simulink library "libH7_3DOF"  (R2021b)
settings: Solver=VariableStepAuto  StartTime=0.0  StopTime=10.0  RelTol=1e-3
undefined symbols (not defined in the file or in its folder): initial_conds, pod
libraries: $bdroot x1
settings Model: Creator=Ferran  LastModifiedBy=Ferran

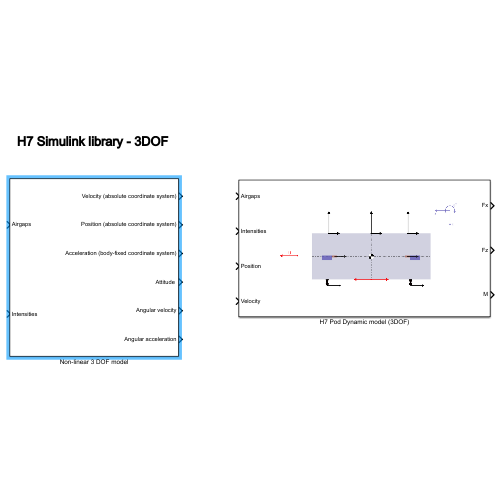
[thumbnail: Simulink's stored preview of the top-level diagram]
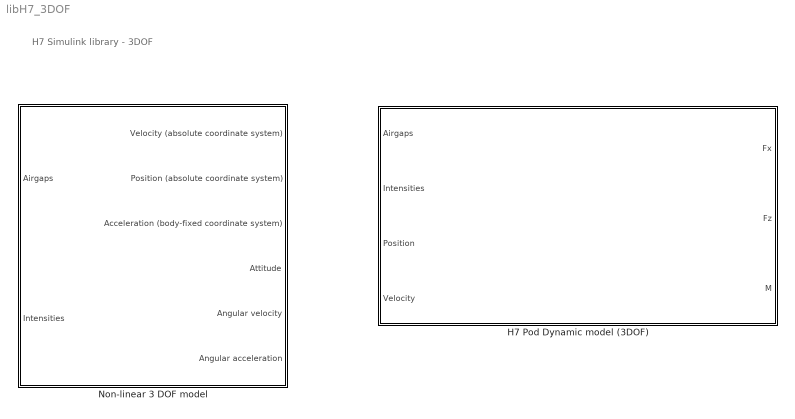
== system libH7_3DOF ==
  note: H7 Simulink library - 3DOF
  H7 Pod Dynamic model (3DOF) : Subsystem
      mask Display: image('FBD_2D.png', [0.12 0.12 0.78 0.78]); % Use "Edit Image" on toolstrip to change.
  Non-linear 3 DOF model : Subsystem

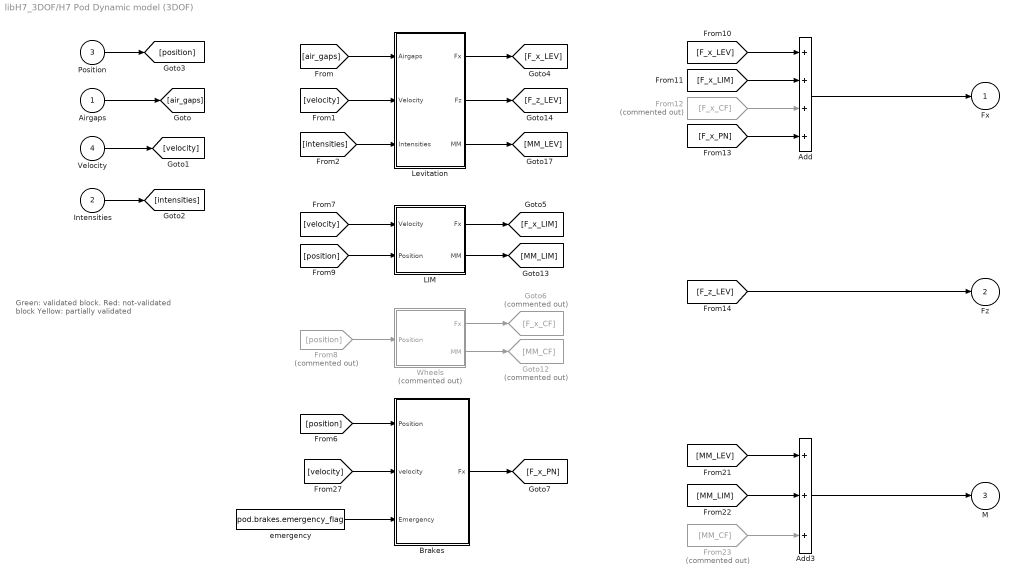
== system libH7_3DOF/H7 Pod Dynamic model (3DOF) ==
  note: Green: validated block.
      | Red: not-validated block
      | Yellow: partially validated
  Airgaps : Inport
  Intensities : Inport  Port=2
  Position : Inport  Port=3
  Velocity : Inport  Port=4
  Add : Sum  Inputs=++++
  Add3 : Sum  Inputs=+++
  "Brakes " : Subsystem  AncestorBlock=libH7/H7 Pod Dynamic model/Brakes
  From12 : From  Commented=on  GotoTag=F_x_CF
  From23 : From  Commented=on  GotoTag=MM_CF
  From8 : From  Commented=on  GotoTag=position
  Goto12 : Goto  Commented=on  GotoTag=MM_CF
  Goto6 : Goto  Commented=on  GotoTag=F_x_CF
  "LIM " : Subsystem  AncestorBlock=libH7/H7 Pod Dynamic model/LIM
  "Levitation " : Subsystem  AncestorBlock=libH7/H7 Pod Dynamic model/Levitation
  "Wheels " : Subsystem  Commented=on  AncestorBlock=libH7/H7 Pod Dynamic model/Wheels
  emergency : Constant  Value=pod.brakes.emergency_flag
  Fx : Outport
  Fz : Outport  Port=2
  M : Outport  Port=3
  wires:
  "Wheels "/2(MM) -> Goto12/1
  "Wheels "/1(Fx) -> Goto6/1
  [velocity] -> "LIM "/1(Velocity)
  [position] -> "Brakes "/1(Position)
  [intensities] -> "Levitation "/3(Intensities)
  [MM_LIM] -> Add3/2
  [velocity] -> "Brakes "/2(velocity)
  Velocity/1 -> [velocity]
  Add3/1 -> M/1
  [velocity] -> "Levitation "/2(Velocity)
  Position/1 -> [position]
  Airgaps/1 -> [air_gaps]
  From8/1 -> "Wheels "/1(Position)
  From23/1 -> Add3/3
  Add/1 -> Fx/1
  [F_x_LIM] -> Add/2
  "Brakes "/1(Fx) -> [F_x_PN]
  [F_x_PN] -> Add/4
  Intensities/1 -> [intensities]
  [F_x_LEV] -> Add/1
  [F_z_LEV] -> Fz/1
  [MM_LEV] -> Add3/1
  "Levitation "/3(MM) -> [MM_LEV]
  [position] -> "LIM "/2(Position)
  "LIM "/2(MM) -> [MM_LIM]
  From12/1 -> Add/3
  "Levitation "/1(Fx) -> [F_x_LEV]
  [air_gaps] -> "Levitation "/1(Airgaps)
  "LIM "/1(Fx) -> [F_x_LIM]
  emergency/1 -> "Brakes "/3(Emergency)
  "Levitation "/2(Fz) -> [F_z_LEV]

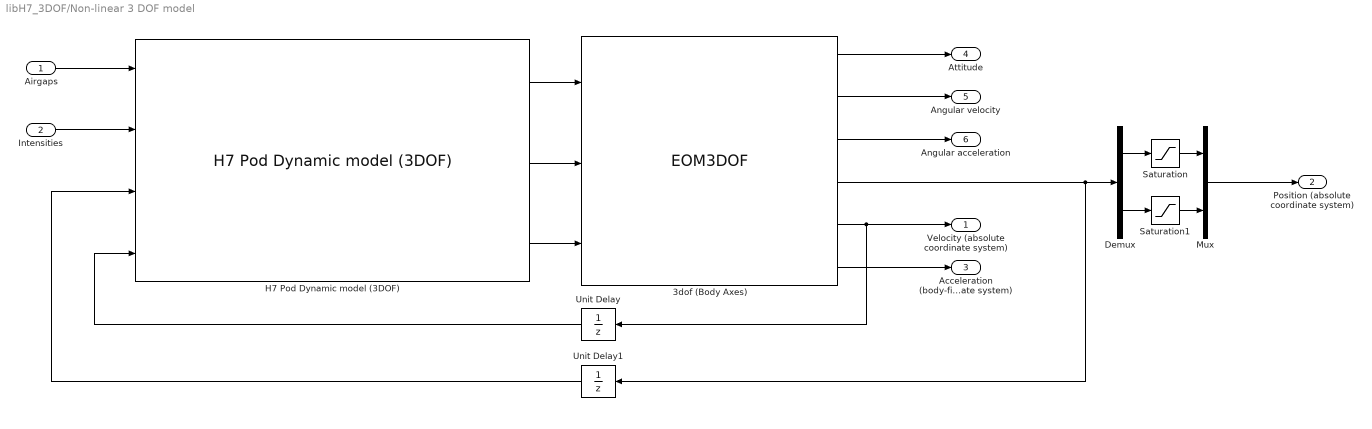
== system libH7_3DOF/Non-linear 3 DOF model ==
  Airgaps : Inport
  Intensities : Inport  Port=2
  3dof (Body Axes) : EOM3DOF  v_ini=1e-10  theta_ini=initial_conds.ang_0(2)  q_ini=initial_conds.w_0(2)  pos_ini=initial_conds.x_0(1:2:3)  mass=pod.mass.mass  Iyy=pod.mass.inertia(2,2)
  Demux : Demux  Outputs=2
  H7 Pod Dynamic model (3DOF) : $bdroot/H7 Pod Dynamic model (3DOF)  SystemSampleTime=-1  VariantActivationTime=update diagram  Latency=0  AutoFrameSizeCalculation=off
  Mux : Mux  Inputs=2
  Saturation : Saturate  UpperLimit=20  LowerLimit=0
  Saturation1 : Saturate  UpperLimit=pod.geometry.z_LEV + 0.023  LowerLimit=pod.geometry.z_LEV + 0.012
  Unit Delay : UnitDelay  InitialCondition=[0,0]  SampleTime=-1  HasFrameUpgradeWarning=on
  Unit Delay1 : UnitDelay  InitialCondition=initial_conds.x_0(1:2:3)  SampleTime=-1  HasFrameUpgradeWarning=on
  Velocity (absolute coordinate system) : Outport
  Position (absolute coordinate system) : Outport  Port=2
  Acceleration (body-fixed coordinate system) : Outport  Port=3
  "Attitude " : Outport  Port=4
  Angular velocity : Outport  Port=5
  Angular acceleration : Outport  Port=6
  wires:
  H7 Pod Dynamic model (3DOF)/1 -> 3dof (Body Axes)/1
  3dof (Body Axes)/2 -> Angular velocity/1
  H7 Pod Dynamic model (3DOF)/3 -> 3dof (Body Axes)/3
  H7 Pod Dynamic model (3DOF)/2 -> 3dof (Body Axes)/2
  Intensities/1 -> H7 Pod Dynamic model (3DOF)/2
  Airgaps/1 -> H7 Pod Dynamic model (3DOF)/1
  3dof (Body Axes)/6 -> Acceleration (body-fixed coordinate system)/1
  3dof (Body Axes)/3 -> Angular acceleration/1
  3dof (Body Axes)/5 -> Velocity (absolute coordinate system)/1, Unit Delay/1
  3dof (Body Axes)/4 -> Demux/1, Unit Delay1/1
  3dof (Body Axes)/1 -> "Attitude "/1
  Demux/1 -> Saturation/1
  Demux/2 -> Saturation1/1
  Mux/1 -> Position (absolute coordinate system)/1
  Unit Delay/1 -> H7 Pod Dynamic model (3DOF)/4
  Unit Delay1/1 -> H7 Pod Dynamic model (3DOF)/3
  Saturation/1 -> Mux/1
  Saturation1/1 -> Mux/2

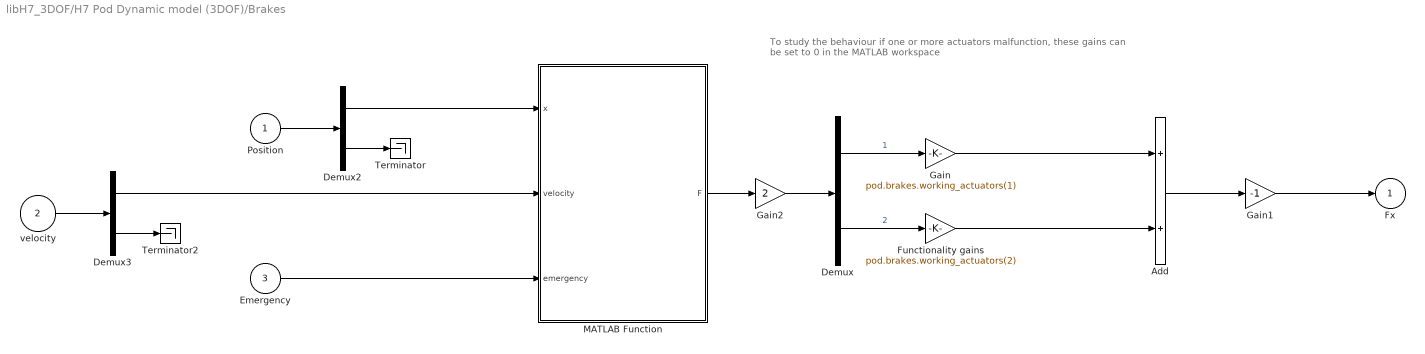
== system libH7_3DOF/H7 Pod Dynamic model (3DOF)/Brakes  ==
  note: To study the behaviour if one or more actuators malfunction,
      | these gains can be set to 0 in the MATLAB workspace
  Position : Inport
  velocity : Inport  Port=2
  Emergency : Inport  Port=3
  Add : Sum
  Demux : Demux  Outputs=2
  Demux2 : Demux  Outputs=2
  Demux3 : Demux  Outputs=2
  Functionality gains : Gain  Gain=pod.brakes.working_actuators(2)
  Gain : Gain  Gain=pod.brakes.working_actuators(1)
  Gain1 : Gain  Gain=-1
  Gain2 : Gain  Gain=2
  MATLAB Function : MATLAB Function  TreatAsAtomicUnit=on
  Terminator : Terminator
  Terminator2 : Terminator
  Fx : Outport
  wires:
  Demux3/1 -> MATLAB Function/2(velocity)
  Demux3/2 -> Terminator2/1
  velocity/1 -> Demux3/1
  Demux2/2 -> Terminator/1
  Demux2/1 -> MATLAB Function/1(x)
  Position/1 -> Demux2/1
  Gain/1 -> Add/1
  Functionality gains/1 -> Add/2
  Demux/2 -> Functionality gains/1  "2"
  Demux/1 -> Gain/1  "1"
  MATLAB Function/1(F) -> Gain2/1
  Emergency/1 -> MATLAB Function/3(emergency)
  Gain2/1 -> Demux/1
  Add/1 -> Gain1/1
  Gain1/1 -> Fx/1

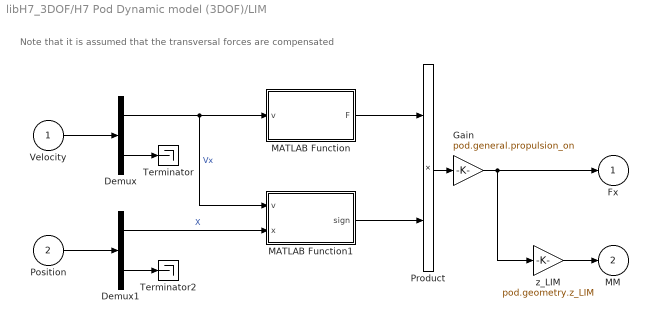
== system libH7_3DOF/H7 Pod Dynamic model (3DOF)/LIM  ==
  note: Note that it is assumed that the transversal forces are compensated
  Velocity : Inport
  Position : Inport  Port=2
  Demux : Demux  Outputs=2
  Demux1 : Demux  Outputs=2
  Gain : Gain  Gain=pod.general.propulsion_on
  MATLAB Function : MATLAB Function  TreatAsAtomicUnit=on
  MATLAB Function1 : MATLAB Function  TreatAsAtomicUnit=on
  Product : Product
  Terminator : Terminator
  Terminator2 : Terminator
  z_LIM : Gain  Gain=pod.geometry.z_LIM
  Fx : Outport
  MM : Outport  Port=2
  wires:
  z_LIM/1 -> MM/1
  Product/1 -> Gain/1
  MATLAB Function/1(F) -> Product/1
  MATLAB Function1/1(sign) -> Product/2
  Demux1/1 -> MATLAB Function1/2(x)  "X"
  Demux1/2 -> Terminator2/1
  Position/1 -> Demux1/1
  Demux/1 -> MATLAB Function1/1(v), MATLAB Function/1(v)  "Vx"
  Demux/2 -> Terminator/1
  Velocity/1 -> Demux/1
  Gain/1 -> Fx/1, z_LIM/1

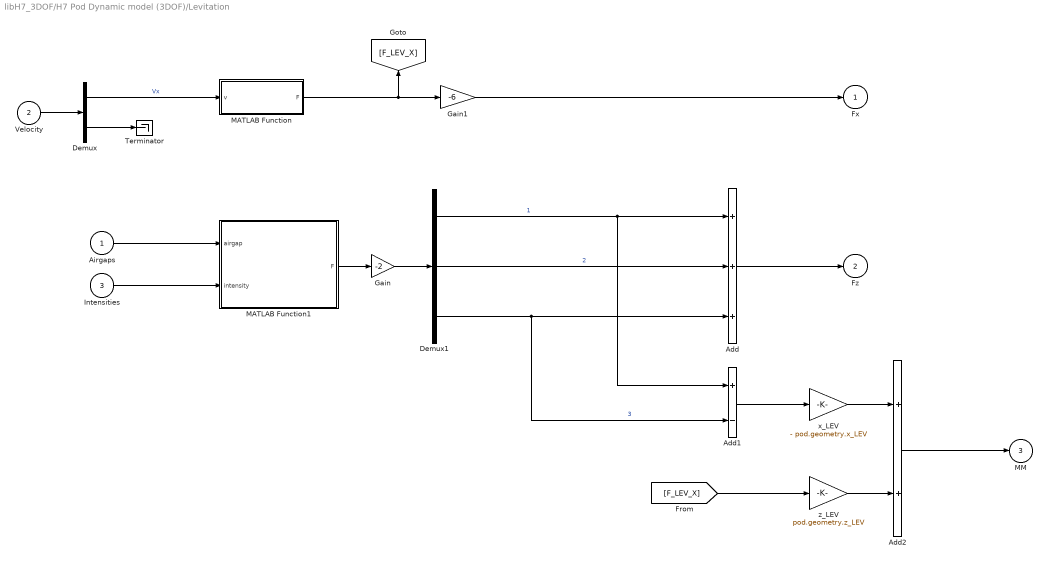
== system libH7_3DOF/H7 Pod Dynamic model (3DOF)/Levitation  ==
  Airgaps : Inport
  Velocity : Inport  Port=2
  Intensities : Inport  Port=3
  Add : Sum  Inputs=+++
  Add1 : Sum  Inputs=+-
  Add2 : Sum
  Demux : Demux  Outputs=2
  Demux1 : Demux  Outputs=3
  Gain : Gain  Gain=-2
  Gain1 : Gain  Gain=-6
  MATLAB Function : MATLAB Function  TreatAsAtomicUnit=on
  MATLAB Function1 : MATLAB Function  TreatAsAtomicUnit=on
  Terminator : Terminator
  x_LEV : Gain  Gain=- pod.geometry.x_LEV
  z_LEV : Gain  Gain=pod.geometry.z_LEV
  Fx : Outport
  Fz : Outport  Port=2
  MM : Outport  Port=3
  wires:
  MATLAB Function/1(F) -> Gain1/1, [F_LEV_X]
  Gain1/1 -> Fx/1
  MATLAB Function1/1(F) -> Gain/1
  Intensities/1 -> MATLAB Function1/2(intensity)
  Airgaps/1 -> MATLAB Function1/1(airgap)
  Demux/1 -> MATLAB Function/1(v)  "Vx"
  Velocity/1 -> Demux/1
  Demux/2 -> Terminator/1
  Gain/1 -> Demux1/1
  Demux1/2 -> Add/2  "2"
  Demux1/3 -> Add1/2, Add/3  "3"
  Demux1/1 -> Add1/1, Add/1  "1"
  Add/1 -> Fz/1
  Add1/1 -> x_LEV/1
  [F_LEV_X] -> z_LEV/1
  z_LEV/1 -> Add2/2
  x_LEV/1 -> Add2/1
  Add2/1 -> MM/1

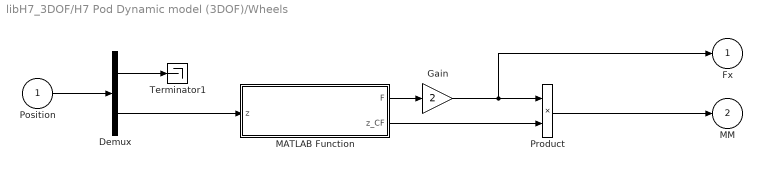
== system libH7_3DOF/H7 Pod Dynamic model (3DOF)/Wheels  ==
  Position : Inport
  Demux : Demux  Outputs=2
  Gain : Gain  Gain=2
  MATLAB Function : MATLAB Function  TreatAsAtomicUnit=on
  Product : Product
  Terminator1 : Terminator
  Fx : Outport
  MM : Outport  Port=2
  wires:
  Product/1 -> MM/1
  MATLAB Function/2(z_CF) -> Product/2
  Demux/1 -> Terminator1/1
  MATLAB Function/1(F) -> Gain/1
  Demux/2 -> MATLAB Function/1(z)
  Position/1 -> Demux/1
  Gain/1 -> Product/1, Fx/1

== matlab function libH7_3DOF/H7 Pod Dynamic model (3DOF)/Brakes /MATLAB Function ==
  data: x input; velocity input; F output; emergency input; pod parameter
function F  = brakes_activation(x, velocity, emergency, pod)
% Computes the braking force of the pneumatic actuators if and only if 
%     (1) The emergency flag has been raised
%     (2) The pod is above the acceleration phase distance
% ═════════════════════════════════════════════════════════════════════════
% Last updated: 20.12.2021
% ═════════════════════════════════════════════════════════════════════════

num_brakes = pod.brakes.n / 2;

if (emergency == 1 && x >= pod.brakes.d && velocity >= 0)
    F       = pod.brakes.force * ones(num_brakes,1);
else
    F       = zeros(num_brakes,1);
end

== matlab function libH7_3DOF/H7 Pod Dynamic model (3DOF)/LIM /MATLAB Function ==
  data: v input; F output; pod parameter
function F = LIMtraction(v, pod)
% Computes the traction force (N) of the LIM as a function of 
% the absolute velocity of the prototype (m/s)
% ═════════════════════════════════════════════════════════════════════════
% Last updated: 20.12.2021
% ═════════════════════════════════════════════════════════════════════════

F = pod.propulsion.poly.p3*v^3 + ...
    pod.propulsion.poly.p2*v^2 + ...
    pod.propulsion.poly.p1*v   + ...
    pod.propulsion.poly.p0;

== matlab function libH7_3DOF/H7 Pod Dynamic model (3DOF)/LIM /MATLAB Function1 ==
  data: v input; x input; sign output; pod parameter
function sign = LIMdirection(v, x, pod)
% Decides if the LIM force is being applied to accelerate or to brake 
% by comparing the position of the pod with a predefined treshold
% ═════════════════════════════════════════════════════════════════════════
% Last updated: 20.12.2021
% ═════════════════════════════════════════════════════════════════════════

if x >= pod.brakes.d && v > 0    
    sign = -1;
elseif x >= pod.brakes.d && v <= 0
    sign = 0;
else
    sign = 1;
end

== matlab function libH7_3DOF/H7 Pod Dynamic model (3DOF)/Levitation /MATLAB Function ==
  data: v input; F output; pod parameter
function F = HEMSdrag(v, pod)
% Computes the drag force (N) of one HEMS unit as a function of the 
% velocity (m/s)
% ═════════════════════════════════════════════════════════════════════════
% Last updated: 16.01.2022
% ═════════════════════════════════════════════════════════════════════════

if v < 1e-3
    v = 0;
end

F = pod.levitation.drag_1_unit.poly.p3*v^3 + ...
    pod.levitation.drag_1_unit.poly.p2*v^2 + ...
    pod.levitation.drag_1_unit.poly.p1*v   + ...
    pod.levitation.drag_1_unit.poly.p0;

== matlab function libH7_3DOF/H7 Pod Dynamic model (3DOF)/Levitation /MATLAB Function1 ==
  data: airgap input; F output; intensity input; pod parameter
function F = HEMSlev(airgap, intensity, pod)
% Computes the levitation force (N) of all the HEMS units as a function of 
% their air gaps (mm) and intensities (A)
% ═════════════════════════════════════════════════════════════════════════
% Last updated: 15.12.2021
% ════════════════════════════════════════════════════════════════════════

x   = airgap;
y   = intensity;

F = pod.levitation.poly_1_unit.p00 + ...
    pod.levitation.poly_1_unit.p10.*x + ...
    pod.levitation.poly_1_unit.p01.*y + ...
    pod.levitation.poly_1_unit.p20.*x.^2 + ...
    pod.levitation.poly_1_unit.p11.*x.*y + ...
    pod.levitation.poly_1_unit.p02.*y.^2 + ...
    pod.levitation.poly_1_unit.p21.*x.^2.*y + ...
    pod.levitation.poly_1_unit.p12.*x.*y.^2 + ...
    pod.levitation.poly_1_unit.p03.*y.^3;

== matlab function libH7_3DOF/H7 Pod Dynamic model (3DOF)/Wheels /MATLAB Function ==
  data: z input; F output; pod parameter; z_CF output
function [F, z_CF] = rollingFriction(z, pod)
% Computes the rolling resistance force (N) of the wheels. It distinguishes
% 3 cases: 
%   (1) z = 0. Pod touching the ground
%   (2) z = z_max. Pod touching the ceiling. It is assumed no current
%   applied to the HEMS. 
%   (3) Otherwise. Pod levitating. 
% ═════════════════════════════════════════════════════════════════════════
% Last updated: 26.12.2021
% ═════════════════════════════════════════════════════════════════════════

% F_LEV worst case scenario computation
x   = 12; % [mm]
y   = 0;  % [A]

F_LEV = pod.levitation.poly_1_unit.p00 + ...
        pod.levitation.poly_1_unit.p10.*x + ...
        pod.levitation.poly_1_unit.p01.*y + ...
        pod.levitation.poly_1_unit.p20.*x.^2 + ...
        pod.levitation.poly_1_unit.p11.*x.*y + ...
        pod.levitation.poly_1_unit.p02.*y.^2 + ...
        pod.levitation.poly_1_unit.p21.*x.^2.*y + ...
        pod.levitation.poly_1_unit.p12.*x.*y.^2 + ...
        pod.levitation.poly_1_unit.p03.*y.^3;

% Main algorithm
if z == 0
    F_N   = pod.mass.mass * 9.81;
    z_CF  = - pod.geometry.z_CF;
elseif z == pod.general.z_range
    F_N   = 6 * F_LEV - pod.mass.mass * 9.81;
    z_CF  = pod.geometry.z_CF;
else
    F_N   = 0;
    z_CF  = 0;
end

F = pod.wheels.number * pod.wheels.roll_coef * F_N;
